simulink model "ImaginaryShort"  (R2015a)
settings: Solver=ode15s  SolverMode=SingleTasking  StartTime=0.0  StopTime=0.01  MaxStep=0.00001  RelTol=1e-3
libraries: fl_lib x7, nesl_utility x4
settings Model: CovMetricSettings=dwe  CovHtmlReporting=off  covSaveCumulativeToWorkspaceVar=off  CovSaveSingleToWorkspaceVar=off  CovExternalEMLEnable=on  Creator=ykamatan  LastModifiedBy=ykamatan
settings SolverCC: ZeroCrossAlgorithm=Adaptive  SolverResetMethod=Robust
settings DataIOCC: LimitDataPoints=off  SaveFormat=Dataset  ReturnWorkspaceOutputs=on
settings DebuggingCC: AlgebraicLoopMsg=none  UnconnectedInputMsg=none  UnconnectedOutputMsg=none  UnconnectedLineMsg=none  SFUnexpectedBacktrackingDiag=error  SFNoUnconditionalDefaultTransitionDiag=error
settings HardwareCC: ProdBitPerPointer=64  ProdLargestAtomicFloat=Float  ProdIntDivRoundTo=Zero  ProdEndianess=LittleEndian  ProdHWDeviceType=Specified
settings ModelReferenceCC: PropagateSignalLabelsOutOfModel=on
settings SFSimCC: SimUseLocalCustomCode=on
settings RTWCC: RTWUseLocalCustomCode=on
settings GRTTargetCC: TargetLangStandard=C99 (ISO)
settings ConfigurationSet: Description=Simscape Multibody

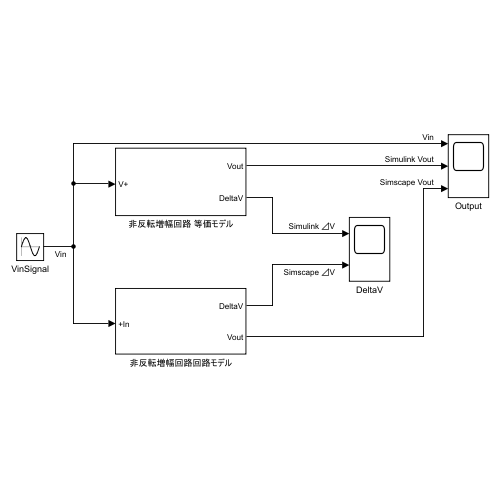
[thumbnail: Simulink's stored preview of the top-level diagram]
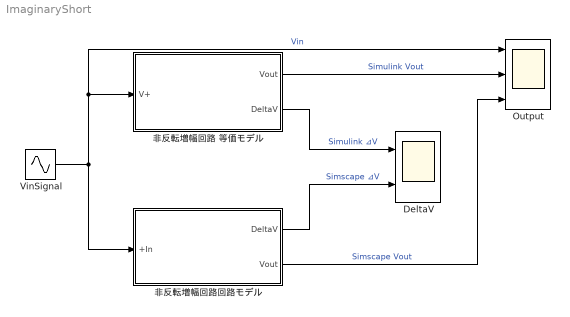
== system ImaginaryShort ==
  DeltaV : Scope  NumInputPorts=2
      settings: TimeRange=auto  ShowLegends=on  MaxDataPoints=5000  SaveToWorkspace=off  YMin=-1~-5  YMax=1~5  SampleTime=-1
  Output : Scope  NumInputPorts=3
      settings: TimeRange=auto  ShowLegends=on  MaxDataPoints=5000  SaveToWorkspace=off  SaveName=ScopeData  YMin=-4.12494~-8.24823~-5  YMax=4.12494~8.24823~5  SampleTime=-1
  VinSignal : Sin  Amplitude=3.3  Frequency=2*pi*440  SampleTime=0
  非反転増幅回路 等価モデル : Subsystem
  非反転増幅回路回路モデル : Subsystem
  wires:
  VinSignal/1 -> Output/1, 非反転増幅回路 等価モデル/1(V+), 非反転増幅回路回路モデル/1(+In)  "Vin"
  非反転増幅回路 等価モデル/1(Vout) -> Output/2  "Simulink Vout"
  非反転増幅回路回路モデル/2(Vout) -> Output/3  "Simscape Vout"
  非反転増幅回路回路モデル/1(DeltaV) -> DeltaV/2  "Simscape ⊿V"
  非反転増幅回路 等価モデル/2(DeltaV) -> DeltaV/1  "Simulink ⊿V"

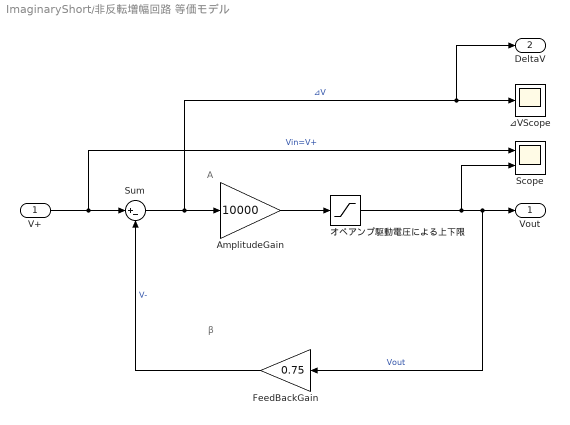
== system ImaginaryShort/非反転増幅回路 等価モデル ==
  note: β
  note: A
  V+ : Inport
  AmplitudeGain : Gain  Gain=10000
  FeedBackGain : Gain  Gain=0.75
  Scope : Scope  NumInputPorts=2
      settings: TimeRange=auto  ShowLegends=on  MaxDataPoints=5000  SaveToWorkspace=off  YMin=-5.49927~-5  YMax=5.49925~5  SampleTime=-1
  Sum : Sum  Inputs=|+-
  ⊿VScope : Scope
      settings: TimeRange=auto  ShowLegends=on  MaxDataPoints=5000  SaveToWorkspace=off  SaveName=ScopeData5  YMin=-0.00055  YMax=0.00055  SampleTime=-1
  オペアンプ駆動電圧による上下限 : Saturate  UpperLimit=15  LowerLimit=-15
      settings: AttributesFormatString=|
      | Max:%<UpperLimit>[V]
      | Min:%<LowerLimit>[V]
  Vout : Outport
  DeltaV : Outport  Port=2
  wires:
  FeedBackGain/1 -> Sum/2  "V-"
  V+/1 -> Scope/1, Sum/1  "Vin=V+"
  Sum/1 -> ⊿VScope/1, DeltaV/1, AmplitudeGain/1  "⊿V"
  AmplitudeGain/1 -> オペアンプ駆動電圧による上下限/1
  オペアンプ駆動電圧による上下限/1 -> FeedBackGain/1, Vout/1, Scope/2  "Vout"

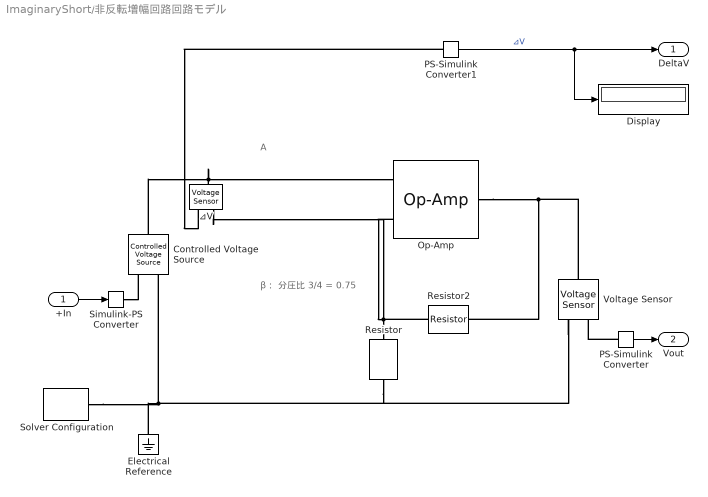
== system ImaginaryShort/非反転増幅回路回路モデル ==
  note: A
  note: β： 分圧比 3/4 = 0.75
  +In : Inport
  Controlled Voltage Source : fl_lib/Electrical/Electrical Sources/Controlled Voltage Source
  Display : Display
  Electrical Reference : fl_lib/Electrical/Electrical Elements/Electrical Reference
  Op-Amp : fl_lib/Electrical/Electrical Elements/Op-Amp  outI_specify=off  outI_priority=None  outI=0 A  outI_nominal_specify=off  outI_nominal_unit=A  outI_nominal_value=1
  PS-Simulink Converter : nesl_utility/PS-Simulink Converter  PhysicalDomain=network_engine_domain  SubClassName=ps_output  LeftPortType=input  RightPortType=output  PseudoPeriodic=off  Frequencies=[]  VectorFormat=inherit  AffineConversion=off
  PS-Simulink Converter1 : nesl_utility/PS-Simulink Converter  PhysicalDomain=network_engine_domain  SubClassName=ps_output  LeftPortType=input  RightPortType=output  PseudoPeriodic=off  Frequencies=[]  VectorFormat=inherit  AffineConversion=off
  Resistor : fl_lib/Electrical/Electrical Elements/Resistor  R=30 MOhm  i_specify=off  i_priority=None  i=0 A  i_nominal_specify=off  i_nominal_unit=A  i_nominal_value=1  v_specify=off  v_priority=None  v=0 V  v_nominal_specify=off  v_nominal_unit=V  v_nominal_value=1
      settings: AttributesFormatString=%<R>%<R_unit>
  Resistor2 : fl_lib/Electrical/Electrical Elements/Resistor  R=10 MOhm  i_specify=off  i_priority=None  i=0 A  i_nominal_specify=off  i_nominal_unit=A  i_nominal_value=1  v_specify=off  v_priority=None  v=0 V  v_nominal_specify=off  v_nominal_unit=V  v_nominal_value=1
      settings: AttributesFormatString=%<R>%<R_unit>
  Simulink-PS Converter : nesl_utility/Simulink-PS Converter  PhysicalDomain=network_engine_domain  SubClassName=ps_input  LeftPortType=input  RightPortType=output  PseudoPeriodic=off  Frequencies=[]  NoiseDistribution=none  NoiseParameters=[]  AffineConversion=off  FilteringAndDerivatives=provide  SimscapeFilterOrder=1  InputFilterTimeConstant=0.001  UdotUserProvided=0
  Solver Configuration : nesl_utility/Solver Configuration  PhysicalDomain=network_engine_domain  SubClassName=solver  LeftPortType=input  RightPortType=generic  Tones=[]  Harmonics=[]  SimulateNoise=off  Profile=off  UseLocalSampling=off  EnableSwitchedLinearOptims=on  FrequencyDomain=off  UseCCode=off  RelTol=0.001  AbsTol=0.001  MinStep=1e-09  ToWorkspace=off  RevertToSquareIcSolve=off  NumHomotopyIterations=100  PhasorMode=off  PhasorModeNumHarmonics=1  ConsistencySolver=NEWTON_XTOL_AFTER_FTOL  IndexReductionMethod=DerivativeReplacement  DoDC=off  ResidualTolerance=1e-09  ConsistencyTolSource=GLOBAL  ConsistencyAbsTol=0.001  ConsistencyRelTol=0.001  ConsistencyTolFactor=0.001  UseLocalSolver=off  LocalSolverChoice=NE_BACKWARD_EULER_ADVANCER  ResolveIndetEquations=on  FunctionEvalNumThread=1  LocalSolverSampleTime=0.001  DoFixedCost=off  MaxNonlinIter=3  MaxModeIter=2  ComputeImpulses=off  ImpulseIterations=2  LinearAlgebra=auto  LinearAlgebraNumThread=0  EquationFormulation=NE_TIME_EF  DelaysMemoryBudget=1024  AutomaticFiltering=on  FilteringTimeConstant=0.001  PartitionStorageMethod=AS_NEEDED  PartitionMemoryBudget=1024  PartitionMethod=ROBUST
  Voltage Sensor : fl_lib/Electrical/Electrical Sensors/Voltage Sensor
  ⊿V : fl_lib/Electrical/Electrical Sensors/Voltage Sensor
  DeltaV : Outport
  Vout : Outport  Port=2
  wires:
  PS-Simulink Converter/1 -> Vout/1
  +In/1 -> Simulink-PS Converter/1
  PS-Simulink Converter1/1 -> DeltaV/1, Display/1  "⊿V"
  connections:
  Resistor2/RConn1 -- Op-Amp/LConn2 -- ⊿V/RConn2 -- Resistor/LConn1
  Electrical Reference/LConn1 -- Voltage Sensor/RConn2 -- Resistor/RConn1 -- Controlled Voltage Source/RConn2 -- Solver Configuration/RConn1
  Op-Amp/RConn1 -- Voltage Sensor/LConn1 -- Resistor2/LConn1
  Controlled Voltage Source/LConn1 -- Op-Amp/LConn1 -- ⊿V/LConn1
  PS-Simulink Converter/LConn1 -- Voltage Sensor/RConn1
  Simulink-PS Converter/RConn1 -- Controlled Voltage Source/RConn1
  PS-Simulink Converter1/LConn1 -- ⊿V/RConn1
